simulink model "fft_512pt_co_sim"  (Simulink 8.0)
settings: Solver=ode45  StartTime=0.0  StopTime=1000  RelTol=1e-3
libraries: xbsIndex_r4 x1077
(part 2 of 2)

== system fft_512pt_co_sim/InputConverter2/dataconv28 ==
  In1 : Inport
   {1..25,27..65} (64 alike) : xbsIndex_r4/Gateway In  gui_display_data_type=Boolean  arith_type=Boolean  n_bits=16  bin_pt=14  preci_type=Single  exp_width=8  frac_width=24  quantization="Round  (unbiased: +/- Inf)"  overflow=Saturate  period=1  dbl_ovrd=off  timing_constraint=None  locs_specified=off  LOCs={}  UseAsADC=off  ADCChannel='1'  inherit_from_input=off  hdl_port=on  block_type=gatewayin
  Concat : xbsIndex_r4/Concat  num_inputs=64  dbl_ovrd=off  block_type=concat
  Demux : Demux  Outputs=64
  Out1 : Outport
  wires:
  Demux/12 -> " 12"/1
  Demux/14 -> " 14"/1
  Demux/15 -> " 15"/1
  Demux/17 -> " 17"/1
  Demux/10 -> " 10"/1
  Demux/16 -> " 16"/1
  Demux/18 -> " 27"/1
  Demux/19 -> " 28"/1
  Demux/7 -> " 7"/1
  Demux/20 -> " 29"/1
  Demux/9 -> " 9"/1
  Demux/2 -> " 2"/1
  Demux/13 -> " 13"/1
  Demux/3 -> " 3"/1
  Demux/6 -> " 6"/1
  Demux/11 -> " 11"/1
  Demux/1 -> " 51"/1
  Demux/8 -> " 8"/1
  Demux/4 -> " 4"/1
  Demux/5 -> " 5"/1
  Demux/21 -> " 30"/1
  Demux/25 -> " 18"/1
  Demux/26 -> " 19"/1
  Demux/22 -> " 31"/1
  Demux/30 -> " 23"/1
  Demux/23 -> " 32"/1
  Demux/24 -> " 33"/1
  Demux/27 -> " 20"/1
  Demux/28 -> " 21"/1
  Demux/31 -> " 24"/1
  Demux/32 -> " 25"/1
  Demux/29 -> " 22"/1
  Demux/36 -> " 61"/1
  Demux/34 -> " 55"/1
  Demux/35 -> " 60"/1
  Demux/33 -> " 44"/1
  Demux/49 -> " 52"/1
  Demux/43 -> " 36"/1
  Demux/42 -> " 35"/1
  Demux/44 -> " 37"/1
  Demux/51 -> " 54"/1
  Demux/59 -> " 46"/1
  Demux/60 -> " 47"/1
  Demux/54 -> " 58"/1
  Demux/61 -> " 48"/1
  Demux/47 -> " 40"/1
  Demux/46 -> " 39"/1
  Demux/55 -> " 59"/1
  Demux/39 -> " 64"/1
  Demux/41 -> " 34"/1
  Demux/58 -> " 45"/1
  Demux/52 -> " 56"/1
  Demux/53 -> " 57"/1
  Demux/56 -> " 42"/1
  Demux/57 -> " 43"/1
  Demux/38 -> " 63"/1
  Demux/62 -> " 49"/1
  Demux/50 -> " 53"/1
  Demux/63 -> " 1"/1
  Demux/40 -> " 65"/1
  Demux/48 -> " 41"/1
  Demux/64 -> " 50"/1
  Demux/45 -> " 38"/1
  Demux/37 -> " 62"/1
  " 13"/1 -> Concat/13
  " 11"/1 -> Concat/11
  " 16"/1 -> Concat/16
  " 15"/1 -> Concat/15
  " 10"/1 -> Concat/10
  " 14"/1 -> Concat/14
  " 12"/1 -> Concat/12
  " 17"/1 -> Concat/17
  " 2"/1 -> Concat/2
  " 3"/1 -> Concat/3
  " 7"/1 -> Concat/7
  " 6"/1 -> Concat/6
  " 9"/1 -> Concat/9
  " 8"/1 -> Concat/8
  " 42"/1 -> Concat/56
  " 35"/1 -> Concat/42
  " 43"/1 -> Concat/57
  " 40"/1 -> Concat/47
  " 36"/1 -> Concat/43
  " 34"/1 -> Concat/41
  " 37"/1 -> Concat/44
  " 38"/1 -> Concat/45
  " 41"/1 -> Concat/48
  " 39"/1 -> Concat/46
  " 52"/1 -> Concat/49
  " 56"/1 -> Concat/52
  " 49"/1 -> Concat/62
  " 1"/1 -> Concat/63
  " 44"/1 -> Concat/33
  " 55"/1 -> Concat/34
  " 54"/1 -> Concat/51
  " 53"/1 -> Concat/50
  " 48"/1 -> Concat/61
  " 46"/1 -> Concat/59
  " 45"/1 -> Concat/58
  " 47"/1 -> Concat/60
  " 63"/1 -> Concat/38
  " 62"/1 -> Concat/37
  " 64"/1 -> Concat/39
  " 60"/1 -> Concat/35
  " 65"/1 -> Concat/40
  " 59"/1 -> Concat/55
  " 58"/1 -> Concat/54
  " 57"/1 -> Concat/53
  " 61"/1 -> Concat/36
  " 19"/1 -> Concat/26
  " 20"/1 -> Concat/27
  " 21"/1 -> Concat/28
  " 22"/1 -> Concat/29
  " 23"/1 -> Concat/30
  " 18"/1 -> Concat/25
  " 24"/1 -> Concat/31
  " 25"/1 -> Concat/32
  " 28"/1 -> Concat/19
  " 27"/1 -> Concat/18
  " 30"/1 -> Concat/21
  " 29"/1 -> Concat/20
  " 31"/1 -> Concat/22
  " 32"/1 -> Concat/23
  " 33"/1 -> Concat/24
  " 4"/1 -> Concat/4
  " 5"/1 -> Concat/5
  " 50"/1 -> Concat/64
  " 51"/1 -> Concat/1
  In1/1 -> Demux/1
  Concat/1 -> Out1/1

== system fft_512pt_co_sim/InputConverter2/dataconv29 ==
  In1 : Inport
   {1..25,27..65} (64 alike) : xbsIndex_r4/Gateway In  gui_display_data_type=Boolean  arith_type=Boolean  n_bits=16  bin_pt=14  preci_type=Single  exp_width=8  frac_width=24  quantization="Round  (unbiased: +/- Inf)"  overflow=Saturate  period=1  dbl_ovrd=off  timing_constraint=None  locs_specified=off  LOCs={}  UseAsADC=off  ADCChannel='1'  inherit_from_input=off  hdl_port=on  block_type=gatewayin
  Concat : xbsIndex_r4/Concat  num_inputs=64  dbl_ovrd=off  block_type=concat
  Demux : Demux  Outputs=64
  Out1 : Outport
  wires:
  Demux/12 -> " 12"/1
  Demux/14 -> " 14"/1
  Demux/15 -> " 15"/1
  Demux/17 -> " 17"/1
  Demux/10 -> " 10"/1
  Demux/16 -> " 16"/1
  Demux/18 -> " 27"/1
  Demux/19 -> " 28"/1
  Demux/7 -> " 7"/1
  Demux/20 -> " 29"/1
  Demux/9 -> " 9"/1
  Demux/2 -> " 2"/1
  Demux/13 -> " 13"/1
  Demux/3 -> " 3"/1
  Demux/6 -> " 6"/1
  Demux/11 -> " 11"/1
  Demux/1 -> " 51"/1
  Demux/8 -> " 8"/1
  Demux/4 -> " 4"/1
  Demux/5 -> " 5"/1
  Demux/21 -> " 30"/1
  Demux/25 -> " 18"/1
  Demux/26 -> " 19"/1
  Demux/22 -> " 31"/1
  Demux/30 -> " 23"/1
  Demux/23 -> " 32"/1
  Demux/24 -> " 33"/1
  Demux/27 -> " 20"/1
  Demux/28 -> " 21"/1
  Demux/31 -> " 24"/1
  Demux/32 -> " 25"/1
  Demux/29 -> " 22"/1
  Demux/36 -> " 61"/1
  Demux/34 -> " 55"/1
  Demux/35 -> " 60"/1
  Demux/33 -> " 44"/1
  Demux/49 -> " 52"/1
  Demux/43 -> " 36"/1
  Demux/42 -> " 35"/1
  Demux/44 -> " 37"/1
  Demux/51 -> " 54"/1
  Demux/59 -> " 46"/1
  Demux/60 -> " 47"/1
  Demux/54 -> " 58"/1
  Demux/61 -> " 48"/1
  Demux/47 -> " 40"/1
  Demux/46 -> " 39"/1
  Demux/55 -> " 59"/1
  Demux/39 -> " 64"/1
  Demux/41 -> " 34"/1
  Demux/58 -> " 45"/1
  Demux/52 -> " 56"/1
  Demux/53 -> " 57"/1
  Demux/56 -> " 42"/1
  Demux/57 -> " 43"/1
  Demux/38 -> " 63"/1
  Demux/62 -> " 49"/1
  Demux/50 -> " 53"/1
  Demux/63 -> " 1"/1
  Demux/40 -> " 65"/1
  Demux/48 -> " 41"/1
  Demux/64 -> " 50"/1
  Demux/45 -> " 38"/1
  Demux/37 -> " 62"/1
  " 13"/1 -> Concat/13
  " 11"/1 -> Concat/11
  " 16"/1 -> Concat/16
  " 15"/1 -> Concat/15
  " 10"/1 -> Concat/10
  " 14"/1 -> Concat/14
  " 12"/1 -> Concat/12
  " 17"/1 -> Concat/17
  " 2"/1 -> Concat/2
  " 3"/1 -> Concat/3
  " 7"/1 -> Concat/7
  " 6"/1 -> Concat/6
  " 9"/1 -> Concat/9
  " 8"/1 -> Concat/8
  " 42"/1 -> Concat/56
  " 35"/1 -> Concat/42
  " 43"/1 -> Concat/57
  " 40"/1 -> Concat/47
  " 36"/1 -> Concat/43
  " 34"/1 -> Concat/41
  " 37"/1 -> Concat/44
  " 38"/1 -> Concat/45
  " 41"/1 -> Concat/48
  " 39"/1 -> Concat/46
  " 52"/1 -> Concat/49
  " 56"/1 -> Concat/52
  " 49"/1 -> Concat/62
  " 1"/1 -> Concat/63
  " 44"/1 -> Concat/33
  " 55"/1 -> Concat/34
  " 54"/1 -> Concat/51
  " 53"/1 -> Concat/50
  " 48"/1 -> Concat/61
  " 46"/1 -> Concat/59
  " 45"/1 -> Concat/58
  " 47"/1 -> Concat/60
  " 63"/1 -> Concat/38
  " 62"/1 -> Concat/37
  " 64"/1 -> Concat/39
  " 60"/1 -> Concat/35
  " 65"/1 -> Concat/40
  " 59"/1 -> Concat/55
  " 58"/1 -> Concat/54
  " 57"/1 -> Concat/53
  " 61"/1 -> Concat/36
  " 19"/1 -> Concat/26
  " 20"/1 -> Concat/27
  " 21"/1 -> Concat/28
  " 22"/1 -> Concat/29
  " 23"/1 -> Concat/30
  " 18"/1 -> Concat/25
  " 24"/1 -> Concat/31
  " 25"/1 -> Concat/32
  " 28"/1 -> Concat/19
  " 27"/1 -> Concat/18
  " 30"/1 -> Concat/21
  " 29"/1 -> Concat/20
  " 31"/1 -> Concat/22
  " 32"/1 -> Concat/23
  " 33"/1 -> Concat/24
  " 4"/1 -> Concat/4
  " 5"/1 -> Concat/5
  " 50"/1 -> Concat/64
  " 51"/1 -> Concat/1
  In1/1 -> Demux/1
  Concat/1 -> Out1/1

== system fft_512pt_co_sim/InputConverter2/dataconv3 ==
  In1 : Inport
   {1..25,27..65} (64 alike) : xbsIndex_r4/Gateway In  gui_display_data_type=Boolean  arith_type=Boolean  n_bits=16  bin_pt=14  preci_type=Single  exp_width=8  frac_width=24  quantization="Round  (unbiased: +/- Inf)"  overflow=Saturate  period=1  dbl_ovrd=off  timing_constraint=None  locs_specified=off  LOCs={}  UseAsADC=off  ADCChannel='1'  inherit_from_input=off  hdl_port=on  block_type=gatewayin
  Concat : xbsIndex_r4/Concat  num_inputs=64  dbl_ovrd=off  block_type=concat
  Demux : Demux  Outputs=64
  Out1 : Outport
  wires:
  Demux/12 -> " 12"/1
  Demux/14 -> " 14"/1
  Demux/15 -> " 15"/1
  Demux/17 -> " 17"/1
  Demux/10 -> " 10"/1
  Demux/16 -> " 16"/1
  Demux/18 -> " 27"/1
  Demux/19 -> " 28"/1
  Demux/7 -> " 7"/1
  Demux/20 -> " 29"/1
  Demux/9 -> " 9"/1
  Demux/2 -> " 2"/1
  Demux/13 -> " 13"/1
  Demux/3 -> " 3"/1
  Demux/6 -> " 6"/1
  Demux/11 -> " 11"/1
  Demux/1 -> " 51"/1
  Demux/8 -> " 8"/1
  Demux/4 -> " 4"/1
  Demux/5 -> " 5"/1
  Demux/21 -> " 30"/1
  Demux/25 -> " 18"/1
  Demux/26 -> " 19"/1
  Demux/22 -> " 31"/1
  Demux/30 -> " 23"/1
  Demux/23 -> " 32"/1
  Demux/24 -> " 33"/1
  Demux/27 -> " 20"/1
  Demux/28 -> " 21"/1
  Demux/31 -> " 24"/1
  Demux/32 -> " 25"/1
  Demux/29 -> " 22"/1
  Demux/36 -> " 61"/1
  Demux/34 -> " 55"/1
  Demux/35 -> " 60"/1
  Demux/33 -> " 44"/1
  Demux/49 -> " 52"/1
  Demux/43 -> " 36"/1
  Demux/42 -> " 35"/1
  Demux/44 -> " 37"/1
  Demux/51 -> " 54"/1
  Demux/59 -> " 46"/1
  Demux/60 -> " 47"/1
  Demux/54 -> " 58"/1
  Demux/61 -> " 48"/1
  Demux/47 -> " 40"/1
  Demux/46 -> " 39"/1
  Demux/55 -> " 59"/1
  Demux/39 -> " 64"/1
  Demux/41 -> " 34"/1
  Demux/58 -> " 45"/1
  Demux/52 -> " 56"/1
  Demux/53 -> " 57"/1
  Demux/56 -> " 42"/1
  Demux/57 -> " 43"/1
  Demux/38 -> " 63"/1
  Demux/62 -> " 49"/1
  Demux/50 -> " 53"/1
  Demux/63 -> " 1"/1
  Demux/40 -> " 65"/1
  Demux/48 -> " 41"/1
  Demux/64 -> " 50"/1
  Demux/45 -> " 38"/1
  Demux/37 -> " 62"/1
  " 13"/1 -> Concat/13
  " 11"/1 -> Concat/11
  " 16"/1 -> Concat/16
  " 15"/1 -> Concat/15
  " 10"/1 -> Concat/10
  " 14"/1 -> Concat/14
  " 12"/1 -> Concat/12
  " 17"/1 -> Concat/17
  " 2"/1 -> Concat/2
  " 3"/1 -> Concat/3
  " 7"/1 -> Concat/7
  " 6"/1 -> Concat/6
  " 9"/1 -> Concat/9
  " 8"/1 -> Concat/8
  " 42"/1 -> Concat/56
  " 35"/1 -> Concat/42
  " 43"/1 -> Concat/57
  " 40"/1 -> Concat/47
  " 36"/1 -> Concat/43
  " 34"/1 -> Concat/41
  " 37"/1 -> Concat/44
  " 38"/1 -> Concat/45
  " 41"/1 -> Concat/48
  " 39"/1 -> Concat/46
  " 52"/1 -> Concat/49
  " 56"/1 -> Concat/52
  " 49"/1 -> Concat/62
  " 1"/1 -> Concat/63
  " 44"/1 -> Concat/33
  " 55"/1 -> Concat/34
  " 54"/1 -> Concat/51
  " 53"/1 -> Concat/50
  " 48"/1 -> Concat/61
  " 46"/1 -> Concat/59
  " 45"/1 -> Concat/58
  " 47"/1 -> Concat/60
  " 63"/1 -> Concat/38
  " 62"/1 -> Concat/37
  " 64"/1 -> Concat/39
  " 60"/1 -> Concat/35
  " 65"/1 -> Concat/40
  " 59"/1 -> Concat/55
  " 58"/1 -> Concat/54
  " 57"/1 -> Concat/53
  " 61"/1 -> Concat/36
  " 19"/1 -> Concat/26
  " 20"/1 -> Concat/27
  " 21"/1 -> Concat/28
  " 22"/1 -> Concat/29
  " 23"/1 -> Concat/30
  " 18"/1 -> Concat/25
  " 24"/1 -> Concat/31
  " 25"/1 -> Concat/32
  " 28"/1 -> Concat/19
  " 27"/1 -> Concat/18
  " 30"/1 -> Concat/21
  " 29"/1 -> Concat/20
  " 31"/1 -> Concat/22
  " 32"/1 -> Concat/23
  " 33"/1 -> Concat/24
  " 4"/1 -> Concat/4
  " 5"/1 -> Concat/5
  " 50"/1 -> Concat/64
  " 51"/1 -> Concat/1
  In1/1 -> Demux/1
  Concat/1 -> Out1/1

== system fft_512pt_co_sim/InputConverter2/dataconv7 ==
  In1 : Inport
   {1..25,27..65} (64 alike) : xbsIndex_r4/Gateway In  gui_display_data_type=Boolean  arith_type=Boolean  n_bits=16  bin_pt=14  preci_type=Single  exp_width=8  frac_width=24  quantization="Round  (unbiased: +/- Inf)"  overflow=Saturate  period=1  dbl_ovrd=off  timing_constraint=None  locs_specified=off  LOCs={}  UseAsADC=off  ADCChannel='1'  inherit_from_input=off  hdl_port=on  block_type=gatewayin
  Concat : xbsIndex_r4/Concat  num_inputs=64  dbl_ovrd=off  block_type=concat
  Demux : Demux  Outputs=64
  Out1 : Outport
  wires:
  Demux/12 -> " 12"/1
  Demux/14 -> " 14"/1
  Demux/15 -> " 15"/1
  Demux/17 -> " 17"/1
  Demux/10 -> " 10"/1
  Demux/16 -> " 16"/1
  Demux/18 -> " 27"/1
  Demux/19 -> " 28"/1
  Demux/7 -> " 7"/1
  Demux/20 -> " 29"/1
  Demux/9 -> " 9"/1
  Demux/2 -> " 2"/1
  Demux/13 -> " 13"/1
  Demux/3 -> " 3"/1
  Demux/6 -> " 6"/1
  Demux/11 -> " 11"/1
  Demux/1 -> " 51"/1
  Demux/8 -> " 8"/1
  Demux/4 -> " 4"/1
  Demux/5 -> " 5"/1
  Demux/21 -> " 30"/1
  Demux/25 -> " 18"/1
  Demux/26 -> " 19"/1
  Demux/22 -> " 31"/1
  Demux/30 -> " 23"/1
  Demux/23 -> " 32"/1
  Demux/24 -> " 33"/1
  Demux/27 -> " 20"/1
  Demux/28 -> " 21"/1
  Demux/31 -> " 24"/1
  Demux/32 -> " 25"/1
  Demux/29 -> " 22"/1
  Demux/36 -> " 61"/1
  Demux/34 -> " 55"/1
  Demux/35 -> " 60"/1
  Demux/33 -> " 44"/1
  Demux/49 -> " 52"/1
  Demux/43 -> " 36"/1
  Demux/42 -> " 35"/1
  Demux/44 -> " 37"/1
  Demux/51 -> " 54"/1
  Demux/59 -> " 46"/1
  Demux/60 -> " 47"/1
  Demux/54 -> " 58"/1
  Demux/61 -> " 48"/1
  Demux/47 -> " 40"/1
  Demux/46 -> " 39"/1
  Demux/55 -> " 59"/1
  Demux/39 -> " 64"/1
  Demux/41 -> " 34"/1
  Demux/58 -> " 45"/1
  Demux/52 -> " 56"/1
  Demux/53 -> " 57"/1
  Demux/56 -> " 42"/1
  Demux/57 -> " 43"/1
  Demux/38 -> " 63"/1
  Demux/62 -> " 49"/1
  Demux/50 -> " 53"/1
  Demux/63 -> " 1"/1
  Demux/40 -> " 65"/1
  Demux/48 -> " 41"/1
  Demux/64 -> " 50"/1
  Demux/45 -> " 38"/1
  Demux/37 -> " 62"/1
  " 13"/1 -> Concat/13
  " 11"/1 -> Concat/11
  " 16"/1 -> Concat/16
  " 15"/1 -> Concat/15
  " 10"/1 -> Concat/10
  " 14"/1 -> Concat/14
  " 12"/1 -> Concat/12
  " 17"/1 -> Concat/17
  " 2"/1 -> Concat/2
  " 3"/1 -> Concat/3
  " 7"/1 -> Concat/7
  " 6"/1 -> Concat/6
  " 9"/1 -> Concat/9
  " 8"/1 -> Concat/8
  " 42"/1 -> Concat/56
  " 35"/1 -> Concat/42
  " 43"/1 -> Concat/57
  " 40"/1 -> Concat/47
  " 36"/1 -> Concat/43
  " 34"/1 -> Concat/41
  " 37"/1 -> Concat/44
  " 38"/1 -> Concat/45
  " 41"/1 -> Concat/48
  " 39"/1 -> Concat/46
  " 52"/1 -> Concat/49
  " 56"/1 -> Concat/52
  " 49"/1 -> Concat/62
  " 1"/1 -> Concat/63
  " 44"/1 -> Concat/33
  " 55"/1 -> Concat/34
  " 54"/1 -> Concat/51
  " 53"/1 -> Concat/50
  " 48"/1 -> Concat/61
  " 46"/1 -> Concat/59
  " 45"/1 -> Concat/58
  " 47"/1 -> Concat/60
  " 63"/1 -> Concat/38
  " 62"/1 -> Concat/37
  " 64"/1 -> Concat/39
  " 60"/1 -> Concat/35
  " 65"/1 -> Concat/40
  " 59"/1 -> Concat/55
  " 58"/1 -> Concat/54
  " 57"/1 -> Concat/53
  " 61"/1 -> Concat/36
  " 19"/1 -> Concat/26
  " 20"/1 -> Concat/27
  " 21"/1 -> Concat/28
  " 22"/1 -> Concat/29
  " 23"/1 -> Concat/30
  " 18"/1 -> Concat/25
  " 24"/1 -> Concat/31
  " 25"/1 -> Concat/32
  " 28"/1 -> Concat/19
  " 27"/1 -> Concat/18
  " 30"/1 -> Concat/21
  " 29"/1 -> Concat/20
  " 31"/1 -> Concat/22
  " 32"/1 -> Concat/23
  " 33"/1 -> Concat/24
  " 4"/1 -> Concat/4
  " 5"/1 -> Concat/5
  " 50"/1 -> Concat/64
  " 51"/1 -> Concat/1
  In1/1 -> Demux/1
  Concat/1 -> Out1/1

== system fft_512pt_co_sim/OutputConverter1/512to64 ==
  In1 : Inport
  128to1 : Subsystem
  128to2 : Subsystem
  128to3 : Subsystem
  128to64 : Subsystem
  256to1 : Subsystem
  256to128 : Subsystem
  512to256 : Subsystem
  Out2 : Outport
  Out3 : Outport  Port=2
  Out4 : Outport  Port=3
  Out5 : Outport  Port=4
  Out6 : Outport  Port=5
  Out7 : Outport  Port=6
  Out8 : Outport  Port=7
  Out9 : Outport  Port=8
  wires:
  512to256/1(Out1) -> 256to128/1(In1)
  512to256/2(Out2) -> 256to1/1(In1)
  256to128/1(Out1) -> 128to64/1(In1)
  256to128/2(Out2) -> 128to1/1(In1)
  256to1/1(Out1) -> 128to2/1(In1)
  256to1/2(Out2) -> 128to3/1(In1)
  128to64/1(Out1) -> Out2/1
  128to64/2(Out2) -> Out3/1
  128to1/1(Out1) -> Out4/1
  128to1/2(Out2) -> Out5/1
  128to2/1(Out1) -> Out6/1
  128to2/2(Out2) -> Out7/1
  128to3/1(Out1) -> Out8/1
  128to3/2(Out2) -> Out9/1
  In1/1 -> 512to256/1(In1)

== system fft_512pt_co_sim/OutputConverter2/512to64 ==
  In1 : Inport
  128to1 : Subsystem
  128to2 : Subsystem
  128to3 : Subsystem
  128to64 : Subsystem
  256to1 : Subsystem
  256to128 : Subsystem
  512to256 : Subsystem
  Out2 : Outport
  Out3 : Outport  Port=2
  Out4 : Outport  Port=3
  Out5 : Outport  Port=4
  Out6 : Outport  Port=5
  Out7 : Outport  Port=6
  Out8 : Outport  Port=7
  Out9 : Outport  Port=8
  wires:
  512to256/1(Out1) -> 256to128/1(In1)
  512to256/2(Out2) -> 256to1/1(In1)
  256to128/1(Out1) -> 128to64/1(In1)
  256to128/2(Out2) -> 128to1/1(In1)
  256to1/1(Out1) -> 128to2/1(In1)
  256to1/2(Out2) -> 128to3/1(In1)
  128to64/1(Out1) -> Out2/1
  128to64/2(Out2) -> Out3/1
  128to1/1(Out1) -> Out4/1
  128to1/2(Out2) -> Out5/1
  128to2/1(Out1) -> Out6/1
  128to2/2(Out2) -> Out7/1
  128to3/1(Out1) -> Out8/1
  128to3/2(Out2) -> Out9/1
  In1/1 -> 512to256/1(In1)

== system fft_512pt_co_sim/OutputConverter1/512to64/128to1 ==
  In1 : Inport
  BitBasher : xbsIndex_r4/BitBasher  bitexpr=|  display_expr=off  sr_1=1  arith_type1=Unsigned  bin_pt1=0  sr_2=2  arith_type2=Unsigned  bin_pt2=0  sr_3=3  arith_type3=Unsigned  bin_pt3=0  sr_4=4  arith_type4=Unsigned  bin_pt4=0  dbl_ovrd=off  block_type=bitbasher
      | <!DOCTYPE HTML PUBLIC "-//W3C//DTD HTML 4.0//EN" "http://www.w3.org/TR/REC-html40/strict.dtd">
      | <html><head><meta name="qrichtext" content="1" /><style type="text/css">
      | p, li { white-space: pre-wrap; }
      | </style></head><body style=" font-family:'SimSun'; font-size:9pt; font-weight:400; font-style:normal;">
      | <p style=" margin-top:12px; margin-bottom:12px; margin-left:0px; margin-right:0px; -qt-block-indent:0; text-indent:0px;"><span style=" font-family:'MS Shell Dlg'; font-size:8pt;">a1={b[127:64]}<br />a2={b[63:0]}</span></p></body></html>
  Out1 : Outport
  Out2 : Outport  Port=2
  wires:
  In1/1 -> BitBasher/1
  BitBasher/1 -> Out1/1
  BitBasher/2 -> Out2/1

== system fft_512pt_co_sim/OutputConverter1/512to64/128to2 ==
  In1 : Inport
  BitBasher : xbsIndex_r4/BitBasher  bitexpr=|  display_expr=off  sr_1=1  arith_type1=Unsigned  bin_pt1=0  sr_2=2  arith_type2=Unsigned  bin_pt2=0  sr_3=3  arith_type3=Unsigned  bin_pt3=0  sr_4=4  arith_type4=Unsigned  bin_pt4=0  dbl_ovrd=off  block_type=bitbasher
      | <!DOCTYPE HTML PUBLIC "-//W3C//DTD HTML 4.0//EN" "http://www.w3.org/TR/REC-html40/strict.dtd">
      | <html><head><meta name="qrichtext" content="1" /><style type="text/css">
      | p, li { white-space: pre-wrap; }
      | </style></head><body style=" font-family:'SimSun'; font-size:9pt; font-weight:400; font-style:normal;">
      | <p style=" margin-top:12px; margin-bottom:12px; margin-left:0px; margin-right:0px; -qt-block-indent:0; text-indent:0px;"><span style=" font-family:'MS Shell Dlg'; font-size:8pt;">a1={b[127:64]}<br />a2={b[63:0]}</span></p></body></html>
  Out1 : Outport
  Out2 : Outport  Port=2
  wires:
  In1/1 -> BitBasher/1
  BitBasher/1 -> Out1/1
  BitBasher/2 -> Out2/1

== system fft_512pt_co_sim/OutputConverter1/512to64/128to3 ==
  In1 : Inport
  BitBasher : xbsIndex_r4/BitBasher  bitexpr=|  display_expr=off  sr_1=1  arith_type1=Unsigned  bin_pt1=0  sr_2=2  arith_type2=Unsigned  bin_pt2=0  sr_3=3  arith_type3=Unsigned  bin_pt3=0  sr_4=4  arith_type4=Unsigned  bin_pt4=0  dbl_ovrd=off  block_type=bitbasher
      | <!DOCTYPE HTML PUBLIC "-//W3C//DTD HTML 4.0//EN" "http://www.w3.org/TR/REC-html40/strict.dtd">
      | <html><head><meta name="qrichtext" content="1" /><style type="text/css">
      | p, li { white-space: pre-wrap; }
      | </style></head><body style=" font-family:'SimSun'; font-size:9pt; font-weight:400; font-style:normal;">
      | <p style=" margin-top:12px; margin-bottom:12px; margin-left:0px; margin-right:0px; -qt-block-indent:0; text-indent:0px;"><span style=" font-family:'MS Shell Dlg'; font-size:8pt;">a1={b[127:64]}<br />a2={b[63:0]}</span></p></body></html>
  Out1 : Outport
  Out2 : Outport  Port=2
  wires:
  In1/1 -> BitBasher/1
  BitBasher/1 -> Out1/1
  BitBasher/2 -> Out2/1

== system fft_512pt_co_sim/OutputConverter1/512to64/128to64 ==
  In1 : Inport
  BitBasher : xbsIndex_r4/BitBasher  bitexpr=|  display_expr=off  sr_1=1  arith_type1=Unsigned  bin_pt1=0  sr_2=2  arith_type2=Unsigned  bin_pt2=0  sr_3=3  arith_type3=Unsigned  bin_pt3=0  sr_4=4  arith_type4=Unsigned  bin_pt4=0  dbl_ovrd=off  block_type=bitbasher
      | <!DOCTYPE HTML PUBLIC "-//W3C//DTD HTML 4.0//EN" "http://www.w3.org/TR/REC-html40/strict.dtd">
      | <html><head><meta name="qrichtext" content="1" /><style type="text/css">
      | p, li { white-space: pre-wrap; }
      | </style></head><body style=" font-family:'SimSun'; font-size:9pt; font-weight:400; font-style:normal;">
      | <p style=" margin-top:12px; margin-bottom:12px; margin-left:0px; margin-right:0px; -qt-block-indent:0; text-indent:0px;"><span style=" font-family:'MS Shell Dlg'; font-size:8pt;">a1={b[127:64]}<br />a2={b[63:0]}</span></p></body></html>
  Out1 : Outport
  Out2 : Outport  Port=2
  wires:
  In1/1 -> BitBasher/1
  BitBasher/1 -> Out1/1
  BitBasher/2 -> Out2/1

== system fft_512pt_co_sim/OutputConverter1/512to64/256to1 ==
  In1 : Inport
  BitBasher : xbsIndex_r4/BitBasher  bitexpr=|  display_expr=off  sr_1=1  arith_type1=Unsigned  bin_pt1=0  sr_2=2  arith_type2=Unsigned  bin_pt2=0  sr_3=3  arith_type3=Unsigned  bin_pt3=0  sr_4=4  arith_type4=Unsigned  bin_pt4=0  dbl_ovrd=off  block_type=bitbasher
      | <!DOCTYPE HTML PUBLIC "-//W3C//DTD HTML 4.0//EN" "http://www.w3.org/TR/REC-html40/strict.dtd">
      | <html><head><meta name="qrichtext" content="1" /><style type="text/css">
      | p, li { white-space: pre-wrap; }
      | </style></head><body style=" font-family:'SimSun'; font-size:9pt; font-weight:400; font-style:normal;">
      | <p style=" margin-top:12px; margin-bottom:12px; margin-left:0px; margin-right:0px; -qt-block-indent:0; text-indent:0px;"><span style=" font-family:'MS Shell Dlg'; font-size:8pt;">a1={b[255:128]}<br />a2={b[127:0]}</span></p></body></html>
  Out1 : Outport
  Out2 : Outport  Port=2
  wires:
  In1/1 -> BitBasher/1
  BitBasher/1 -> Out1/1
  BitBasher/2 -> Out2/1

== system fft_512pt_co_sim/OutputConverter1/512to64/256to128 ==
  In1 : Inport
  BitBasher : xbsIndex_r4/BitBasher  bitexpr=|  display_expr=off  sr_1=1  arith_type1=Unsigned  bin_pt1=0  sr_2=2  arith_type2=Unsigned  bin_pt2=0  sr_3=3  arith_type3=Unsigned  bin_pt3=0  sr_4=4  arith_type4=Unsigned  bin_pt4=0  dbl_ovrd=off  block_type=bitbasher
      | <!DOCTYPE HTML PUBLIC "-//W3C//DTD HTML 4.0//EN" "http://www.w3.org/TR/REC-html40/strict.dtd">
      | <html><head><meta name="qrichtext" content="1" /><style type="text/css">
      | p, li { white-space: pre-wrap; }
      | </style></head><body style=" font-family:'SimSun'; font-size:9pt; font-weight:400; font-style:normal;">
      | <p style=" margin-top:12px; margin-bottom:12px; margin-left:0px; margin-right:0px; -qt-block-indent:0; text-indent:0px;"><span style=" font-family:'MS Shell Dlg'; font-size:8pt;">a1={b[255:128]}<br />a2={b[127:0]}</span></p></body></html>
  Out1 : Outport
  Out2 : Outport  Port=2
  wires:
  In1/1 -> BitBasher/1
  BitBasher/1 -> Out1/1
  BitBasher/2 -> Out2/1

== system fft_512pt_co_sim/OutputConverter1/512to64/512to256 ==
  In1 : Inport
  BitBasher : xbsIndex_r4/BitBasher  bitexpr=|  display_expr=off  sr_1=1  arith_type1=Unsigned  bin_pt1=0  sr_2=2  arith_type2=Unsigned  bin_pt2=0  sr_3=3  arith_type3=Unsigned  bin_pt3=0  sr_4=4  arith_type4=Unsigned  bin_pt4=0  dbl_ovrd=off  block_type=bitbasher
      | <!DOCTYPE HTML PUBLIC "-//W3C//DTD HTML 4.0//EN" "http://www.w3.org/TR/REC-html40/strict.dtd">
      | <html><head><meta name="qrichtext" content="1" /><style type="text/css">
      | p, li { white-space: pre-wrap; }
      | </style></head><body style=" font-family:'SimSun'; font-size:9pt; font-weight:400; font-style:normal;">
      | <p style=" margin-top:12px; margin-bottom:12px; margin-left:0px; margin-right:0px; -qt-block-indent:0; text-indent:0px;"><span style=" font-family:'MS Shell Dlg'; font-size:8pt;">a1={b[511:256]}<br />a2={b[255:0]}</span></p></body></html>
  Out1 : Outport
  Out2 : Outport  Port=2
  wires:
  In1/1 -> BitBasher/1
  BitBasher/1 -> Out1/1
  BitBasher/2 -> Out2/1

== system fft_512pt_co_sim/OutputConverter2/512to64/128to1 ==
  In1 : Inport
  BitBasher : xbsIndex_r4/BitBasher  bitexpr=|  display_expr=off  sr_1=1  arith_type1=Unsigned  bin_pt1=0  sr_2=2  arith_type2=Unsigned  bin_pt2=0  sr_3=3  arith_type3=Unsigned  bin_pt3=0  sr_4=4  arith_type4=Unsigned  bin_pt4=0  dbl_ovrd=off  block_type=bitbasher
      | <!DOCTYPE HTML PUBLIC "-//W3C//DTD HTML 4.0//EN" "http://www.w3.org/TR/REC-html40/strict.dtd">
      | <html><head><meta name="qrichtext" content="1" /><style type="text/css">
      | p, li { white-space: pre-wrap; }
      | </style></head><body style=" font-family:'SimSun'; font-size:9pt; font-weight:400; font-style:normal;">
      | <p style=" margin-top:12px; margin-bottom:12px; margin-left:0px; margin-right:0px; -qt-block-indent:0; text-indent:0px;"><span style=" font-family:'MS Shell Dlg'; font-size:8pt;">a1={b[127:64]}<br />a2={b[63:0]}</span></p></body></html>
  Out1 : Outport
  Out2 : Outport  Port=2
  wires:
  In1/1 -> BitBasher/1
  BitBasher/1 -> Out1/1
  BitBasher/2 -> Out2/1

== system fft_512pt_co_sim/OutputConverter2/512to64/128to2 ==
  In1 : Inport
  BitBasher : xbsIndex_r4/BitBasher  bitexpr=|  display_expr=off  sr_1=1  arith_type1=Unsigned  bin_pt1=0  sr_2=2  arith_type2=Unsigned  bin_pt2=0  sr_3=3  arith_type3=Unsigned  bin_pt3=0  sr_4=4  arith_type4=Unsigned  bin_pt4=0  dbl_ovrd=off  block_type=bitbasher
      | <!DOCTYPE HTML PUBLIC "-//W3C//DTD HTML 4.0//EN" "http://www.w3.org/TR/REC-html40/strict.dtd">
      | <html><head><meta name="qrichtext" content="1" /><style type="text/css">
      | p, li { white-space: pre-wrap; }
      | </style></head><body style=" font-family:'SimSun'; font-size:9pt; font-weight:400; font-style:normal;">
      | <p style=" margin-top:12px; margin-bottom:12px; margin-left:0px; margin-right:0px; -qt-block-indent:0; text-indent:0px;"><span style=" font-family:'MS Shell Dlg'; font-size:8pt;">a1={b[127:64]}<br />a2={b[63:0]}</span></p></body></html>
  Out1 : Outport
  Out2 : Outport  Port=2
  wires:
  In1/1 -> BitBasher/1
  BitBasher/1 -> Out1/1
  BitBasher/2 -> Out2/1

== system fft_512pt_co_sim/OutputConverter2/512to64/128to3 ==
  In1 : Inport
  BitBasher : xbsIndex_r4/BitBasher  bitexpr=|  display_expr=off  sr_1=1  arith_type1=Unsigned  bin_pt1=0  sr_2=2  arith_type2=Unsigned  bin_pt2=0  sr_3=3  arith_type3=Unsigned  bin_pt3=0  sr_4=4  arith_type4=Unsigned  bin_pt4=0  dbl_ovrd=off  block_type=bitbasher
      | <!DOCTYPE HTML PUBLIC "-//W3C//DTD HTML 4.0//EN" "http://www.w3.org/TR/REC-html40/strict.dtd">
      | <html><head><meta name="qrichtext" content="1" /><style type="text/css">
      | p, li { white-space: pre-wrap; }
      | </style></head><body style=" font-family:'SimSun'; font-size:9pt; font-weight:400; font-style:normal;">
      | <p style=" margin-top:12px; margin-bottom:12px; margin-left:0px; margin-right:0px; -qt-block-indent:0; text-indent:0px;"><span style=" font-family:'MS Shell Dlg'; font-size:8pt;">a1={b[127:64]}<br />a2={b[63:0]}</span></p></body></html>
  Out1 : Outport
  Out2 : Outport  Port=2
  wires:
  In1/1 -> BitBasher/1
  BitBasher/1 -> Out1/1
  BitBasher/2 -> Out2/1

== system fft_512pt_co_sim/OutputConverter2/512to64/128to64 ==
  In1 : Inport
  BitBasher : xbsIndex_r4/BitBasher  bitexpr=|  display_expr=off  sr_1=1  arith_type1=Unsigned  bin_pt1=0  sr_2=2  arith_type2=Unsigned  bin_pt2=0  sr_3=3  arith_type3=Unsigned  bin_pt3=0  sr_4=4  arith_type4=Unsigned  bin_pt4=0  dbl_ovrd=off  block_type=bitbasher
      | <!DOCTYPE HTML PUBLIC "-//W3C//DTD HTML 4.0//EN" "http://www.w3.org/TR/REC-html40/strict.dtd">
      | <html><head><meta name="qrichtext" content="1" /><style type="text/css">
      | p, li { white-space: pre-wrap; }
      | </style></head><body style=" font-family:'SimSun'; font-size:9pt; font-weight:400; font-style:normal;">
      | <p style=" margin-top:12px; margin-bottom:12px; margin-left:0px; margin-right:0px; -qt-block-indent:0; text-indent:0px;"><span style=" font-family:'MS Shell Dlg'; font-size:8pt;">a1={b[127:64]}<br />a2={b[63:0]}</span></p></body></html>
  Out1 : Outport
  Out2 : Outport  Port=2
  wires:
  In1/1 -> BitBasher/1
  BitBasher/1 -> Out1/1
  BitBasher/2 -> Out2/1

== system fft_512pt_co_sim/OutputConverter2/512to64/256to1 ==
  In1 : Inport
  BitBasher : xbsIndex_r4/BitBasher  bitexpr=|  display_expr=off  sr_1=1  arith_type1=Unsigned  bin_pt1=0  sr_2=2  arith_type2=Unsigned  bin_pt2=0  sr_3=3  arith_type3=Unsigned  bin_pt3=0  sr_4=4  arith_type4=Unsigned  bin_pt4=0  dbl_ovrd=off  block_type=bitbasher
      | <!DOCTYPE HTML PUBLIC "-//W3C//DTD HTML 4.0//EN" "http://www.w3.org/TR/REC-html40/strict.dtd">
      | <html><head><meta name="qrichtext" content="1" /><style type="text/css">
      | p, li { white-space: pre-wrap; }
      | </style></head><body style=" font-family:'SimSun'; font-size:9pt; font-weight:400; font-style:normal;">
      | <p style=" margin-top:12px; margin-bottom:12px; margin-left:0px; margin-right:0px; -qt-block-indent:0; text-indent:0px;"><span style=" font-family:'MS Shell Dlg'; font-size:8pt;">a1={b[255:128]}<br />a2={b[127:0]}</span></p></body></html>
  Out1 : Outport
  Out2 : Outport  Port=2
  wires:
  In1/1 -> BitBasher/1
  BitBasher/1 -> Out1/1
  BitBasher/2 -> Out2/1

== system fft_512pt_co_sim/OutputConverter2/512to64/256to128 ==
  In1 : Inport
  BitBasher : xbsIndex_r4/BitBasher  bitexpr=|  display_expr=off  sr_1=1  arith_type1=Unsigned  bin_pt1=0  sr_2=2  arith_type2=Unsigned  bin_pt2=0  sr_3=3  arith_type3=Unsigned  bin_pt3=0  sr_4=4  arith_type4=Unsigned  bin_pt4=0  dbl_ovrd=off  block_type=bitbasher
      | <!DOCTYPE HTML PUBLIC "-//W3C//DTD HTML 4.0//EN" "http://www.w3.org/TR/REC-html40/strict.dtd">
      | <html><head><meta name="qrichtext" content="1" /><style type="text/css">
      | p, li { white-space: pre-wrap; }
      | </style></head><body style=" font-family:'SimSun'; font-size:9pt; font-weight:400; font-style:normal;">
      | <p style=" margin-top:12px; margin-bottom:12px; margin-left:0px; margin-right:0px; -qt-block-indent:0; text-indent:0px;"><span style=" font-family:'MS Shell Dlg'; font-size:8pt;">a1={b[255:128]}<br />a2={b[127:0]}</span></p></body></html>
  Out1 : Outport
  Out2 : Outport  Port=2
  wires:
  In1/1 -> BitBasher/1
  BitBasher/1 -> Out1/1
  BitBasher/2 -> Out2/1

== system fft_512pt_co_sim/OutputConverter2/512to64/512to256 ==
  In1 : Inport
  BitBasher : xbsIndex_r4/BitBasher  bitexpr=|  display_expr=off  sr_1=1  arith_type1=Unsigned  bin_pt1=0  sr_2=2  arith_type2=Unsigned  bin_pt2=0  sr_3=3  arith_type3=Unsigned  bin_pt3=0  sr_4=4  arith_type4=Unsigned  bin_pt4=0  dbl_ovrd=off  block_type=bitbasher
      | <!DOCTYPE HTML PUBLIC "-//W3C//DTD HTML 4.0//EN" "http://www.w3.org/TR/REC-html40/strict.dtd">
      | <html><head><meta name="qrichtext" content="1" /><style type="text/css">
      | p, li { white-space: pre-wrap; }
      | </style></head><body style=" font-family:'SimSun'; font-size:9pt; font-weight:400; font-style:normal;">
      | <p style=" margin-top:12px; margin-bottom:12px; margin-left:0px; margin-right:0px; -qt-block-indent:0; text-indent:0px;"><span style=" font-family:'MS Shell Dlg'; font-size:8pt;">a1={b[511:256]}<br />a2={b[255:0]}</span></p></body></html>
  Out1 : Outport
  Out2 : Outport  Port=2
  wires:
  In1/1 -> BitBasher/1
  BitBasher/1 -> Out1/1
  BitBasher/2 -> Out2/1
